simulink model "DC_Motor_Transfer_Function_PI_Control (1)"  (R2023b)
settings: Solver=VariableStepAuto  StartTime=0.0  StopTime=100  RelTol=1e-3
InitFcn:
  | ra = 6.9;
  | la = 41.5e-3;
  | Kt=1.424;
  | Ke=0.96;
  | J = .005;
  | B=0.0099;
libraries: slpidlib x1
settings Model: Creator=ravikrishna_g3  LastModifiedBy=abina

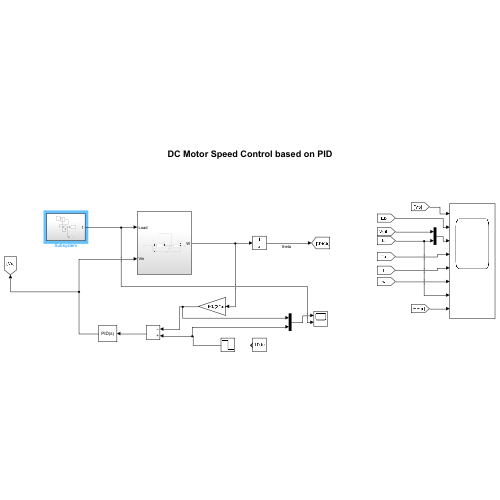
[thumbnail: Simulink's stored preview of the top-level diagram]
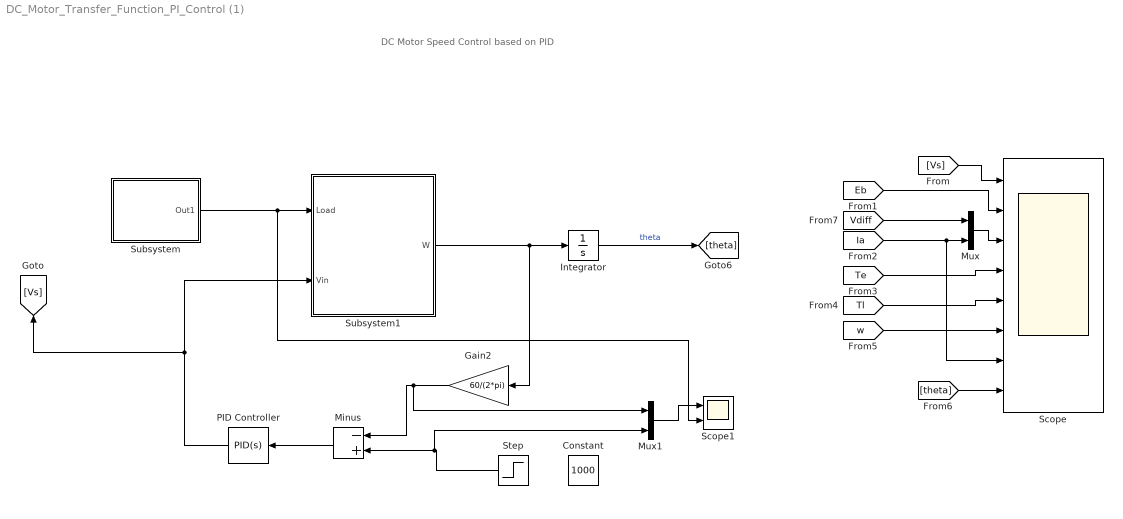
== system DC_Motor_Transfer_Function_PI_Control (1) ==
  note: DC Motor Speed Control based on PID
  Constant : Constant  Value=1000
  Gain2 : Gain  Gain=60/(2*pi)
  Integrator : Integrator
  Minus : Sum  Inputs=-+
  Mux : Mux  Inputs=2
  Mux1 : Mux  Inputs=2
  PID Controller : slpidlib/PID Controller  Controller=PID  Form=Parallel  TimeDomain=Continuous-time  UseExternalTs=off  SampleTime=-1  IntegratorMethod=Forward Euler  FilterMethod=Forward Euler  ControllerParametersSource=internal  P=0.680796727494057  I=31.8708941487701  UseKiTs=off  D=0.00361888997999223  N=27922.8976073358  UseFilter=on  TunerSelectOption=Transfer Function Based (PID Tuner App)  InitialConditionSource=internal  InitialConditionForIntegrator=0  InitialConditionForFilter=0  DifferentiatorICPrevScaledInput=0  ExternalReset=none  TrackingMode=off  Kt=1  LimitOutput=off  SatLimitsSource=internal  UpperSaturationLimit=inf  LowerSaturationLimit=-inf  LinearizeAsGain=on  AntiWindupMode=none  Kb=1  LimitIntegrator=off  UpperIntegratorSaturationLimit=inf  LowerIntegratorSaturationLimit=-inf  POutMin=[]  POutMax=[]  IOutMin=[]  IOutMax=[]  DOutMin=[]  DOutMax=[]  NOutMin=[]  NOutMax=[]  SumOutMin=[]  SumOutMax=[]  SaturationOutMin=[]  SaturationOutMax=[]  PParamMin=[]  PParamMax=[]  IParamMin=[]  IParamMax=[]  DParamMin=[]  DParamMax=[]  NParamMin=[]  NParamMax=[]  KbParamMin=[]  KbParamMax=[]  KtParamMin=[]  KtParamMax=[]  KbOutMin=[]  KbOutMax=[]  KtOutMin=[]  KtOutMax=[]  IntegratorOutMin=[]  IntegratorOutMax=[]  FilterOutMin=[]  FilterOutMax=[]  SumI1OutMin=[]  SumI1OutMax=[]  SumI2OutMin=[]  SumI2OutMax=[]  SumI3OutMin=[]  SumI3OutMax=[]  SumI4OutMin=[]  SumI4OutMax=[]  SumDOutMin=[]  SumDOutMax=[]  DifferentiatorOutMin=[]  DifferentiatorOutMax=[]  FilterDiffOutCoefMin=[]  FilterDiffOutCoefMax=[]  ReciprocalOutMin=[]  ReciprocalOutMax=[]  SumDenOutMin=[]  SumDenOutMax=[]  SumNumOutMin=[]  SumNumOutMax=[]  DivideOutMin=[]  DivideOutMax=[]  UdiffTsProdOutMin=[]  UdiffTsProdOutMax=[]  NTsProdOutMin=[]  NTsProdOutMax=[]  UintegralTsProdOutMin=[]  UintegralTsProdOutMax=[]  UngainTsProdOutMin=[]  UngainTsProdOutMax=[]  ClampingZeroOutDataTypeStr=Inherit: Inherit via back propagation  ClampingZeroOutMin=[]  ClampingZeroOutMax=[]  FilterDenConstantOutDataTypeStr=Inherit: Inherit via back propagation  FilterDenConstantOutMin=[]  FilterDenConstantOutMax=[]  PCopyOutDataTypeStr=Inherit: Inherit via back propagation  PCopyOutMin=[]  PCopyOutMax=[]  NCopyOutDataTypeStr=Inherit: Inherit via back propagation  NCopyOutMin=[]  NCopyOutMax=[]  IntegratorContinuousStateAttributes=''  IntegratorStateMustResolveToSignalObject=off  IntegratorRTWStateStorageClass=Auto  FilterContinuousStateAttributes=''  FilterStateMustResolveToSignalObject=off  FilterRTWStateStorageClass=Auto  ParallelPVariant=InternalParameters  IdealPVariant=Disabled  IVariant=InternalParameters  DVariant=InternalParameters  IntegratorVariant=Continuous  SatVariant=Disabled  AWVariant=Passthrough  PCopyVariant=Disabled  TRVariant=Disabled  FdbkBlocksVariant=Forward  IdealPFdbkVariant=Disabled  SatFdbkVariant=Disabled  DerivativeFilterVariant=ContFilter  NVariant=InternalParameters  NCopyVariant=Disabled  FilterICVariant=InternalICsFilter  IntegratorICVariant=InternalICs  ExternalResetVariant=Disabled  TRSumVariant=Passthrough  SumFdbkVariant=Disabled  SumVariant=Sum_PID  TsampFilterVariant=InternalTs  TsampNgainVariant=Passthrough  TsampIntegralVariant=Disabled_SignalSpec  ExternalSaturationOutDataTypeStr=Inherit: Same as second input
  Scope : Scope  NumInputPorts=8
  Scope1 : Scope  NumInputPorts=2
  Step : Step  Time=50  Before=1200  After=1000  SampleTime=0
  Subsystem : Subsystem
  Subsystem1 : Subsystem
  wires:
  Integrator/1 -> [theta]  "theta"
  [Vs] -> Scope/1
  [Eb] -> Scope/2
  [Ia] -> Mux/2, Scope/7
  [Te] -> Scope/4
  [Tl] -> Scope/5
  [w] -> Scope/6
  [theta] -> Scope/8
  [Vdiff] -> Mux/1
  Mux/1 -> Scope/3
  Subsystem/1(Out1) -> Scope1/2, Subsystem1/1(Load)
  Subsystem1/1(W) -> Gain2/1, Integrator/1
  Gain2/1 -> Mux1/1, Minus/1
  Minus/1 -> PID Controller/1
  PID Controller/1 -> [Vs], Subsystem1/2(Vin)
  Mux1/1 -> Scope1/1
  Step/1 -> Mux1/2, Minus/2

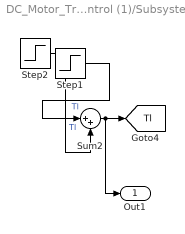
== system DC_Motor_Transfer_Function_PI_Control (1)/Subsystem ==
  Step1 : Step  Time=20  After=5  SampleTime=0
  Step2 : Step  Time=40  After=9  SampleTime=0
  Sum2 : Sum  Inputs=|++
  Out1 : Outport
  tag scope: Tl=global
  wires:
  Sum2/1 -> Out1/1, [Tl]
  Step1/1 -> Sum2/1  "Tl"
  Step2/1 -> Sum2/2  "Tl"

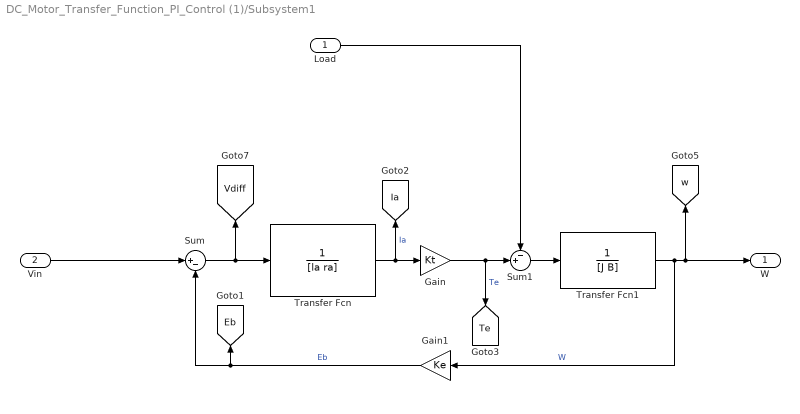
== system DC_Motor_Transfer_Function_PI_Control (1)/Subsystem1 ==
  Load : Inport
  Vin : Inport  Port=2
  Gain : Gain  Gain=Kt
  Gain1 : Gain  Gain=Ke
  Sum : Sum  Inputs=|+-
  Sum1 : Sum  Inputs=-+|
  Transfer Fcn : TransferFcn  Denominator=[la ra]
  Transfer Fcn1 : TransferFcn  Denominator=[J B]
  W : Outport
  tag scope: Eb=global, Ia=global, Te=global, Vdiff=global, w=global
  wires:
  Transfer Fcn/1 -> [Ia], Gain/1  "Ia"
  Gain/1 -> Sum1/2, [Te]  "Te"
  Transfer Fcn1/1 -> W/1, [w], Gain1/1  "W"
  Gain1/1 -> [Eb], Sum/2  "Eb"
  Sum/1 -> [Vdiff], Transfer Fcn/1
  Sum1/1 -> Transfer Fcn1/1
  Vin/1 -> Sum/1
  Load/1 -> Sum1/1
